simulink model "three_phase_harmonics_pll"  (Simulink 10.3)
settings: Solver=ode23tb  StartTime=0.0  StopTime=0.12  FixedStep=1e-6  MaxStep=1e-4  MinStep=1e-5  RelTol=1e-3  EnableMultiTasking=on
libraries: powerlib_extras x1
settings Model: Creator=ankush  LastModifiedBy=HP
settings DataIOCC: LimitDataPoints=on
settings DebuggingCC: SolverPrmCheckMsg=warning

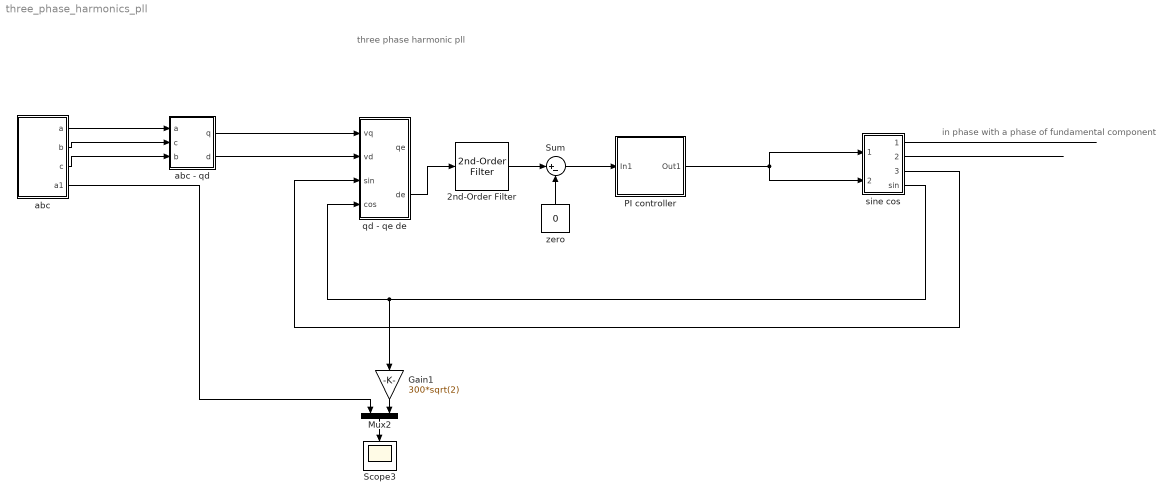
== system three_phase_harmonics_pll ==
  note: in phase with a phase of fundamental component
  note: three phase harmonic pll
  2nd-Order Filter : powerlib_extras/Control  Blocks/2nd-Order Filter  FilterType=Lowpass  Fo=75  Zeta=0.707  Initialize=off  Vac_Init=[1 45 60]  Vdc_Init=-0.5  PlotResponse=off  param1=[1 500 1]
      settings: SourceProductBaseCode=PS
  Gain1 : Gain  Gain=300*sqrt(2)
  Mux2 : Mux  Inputs=2
  PI controller : Subsystem
  Scope3 : Scope
  Sum : Sum  Inputs=|+-
  abc : Subsystem
  abc - qd : Subsystem
  qd - qe de : Subsystem
  sine cos : Subsystem
  zero : Constant  Value=0
  wires:
  abc - qd/1(q) -> qd - qe de/1(vq)
  abc - qd/2(d) -> qd - qe de/2(vd)
  zero/1 -> Sum/2
  sine cos/3(cos) -> qd - qe de/3(sin)
  sine cos/4(sin) -> qd - qe de/4(cos), Gain1/1
  Sum/1 -> PI controller/1(In1)
  PI controller/1(Out1) -> sine cos/1(In1), sine cos/2(In2)
  Mux2/1 -> Scope3/1
  Gain1/1 -> Mux2/2
  abc/2(b) -> abc - qd/2(c)
  abc/1(a) -> abc - qd/1(a)
  abc/3(c) -> abc - qd/3(b)
  qd - qe de/2(de) -> 2nd-Order Filter/1
  2nd-Order Filter/1 -> Sum/1
  abc/4(a1) -> Mux2/1
  sine cos/1(sin1) -> ?
  sine cos/2(cos1) -> ?

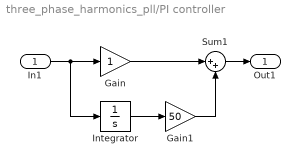
== system three_phase_harmonics_pll/PI controller ==
  In1 : Inport
  Gain : Gain
  Gain1 : Gain  Gain=50
  Integrator : Integrator
  Sum1 : Sum  Inputs=|++
  Out1 : Outport
  wires:
  In1/1 -> Integrator/1, Gain/1
  Integrator/1 -> Gain1/1
  Gain/1 -> Sum1/1
  Gain1/1 -> Sum1/2
  Sum1/1 -> Out1/1

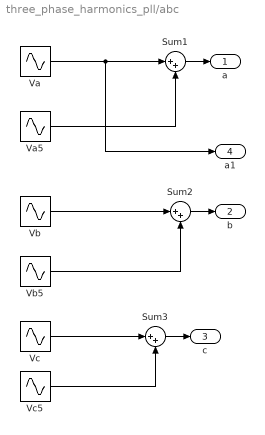
== system three_phase_harmonics_pll/abc ==
  Sum1 : Sum  Inputs=|++
  Sum2 : Sum  Inputs=|++
  Sum3 : Sum  Inputs=|++
  Va : Sin  Amplitude=240*sqrt(2)  Frequency=2*pi*50  SampleTime=0
  Va5 : Sin  Amplitude=50*sqrt(2)  Frequency=2*pi*50*5  SampleTime=0
  Vb : Sin  Amplitude=240*sqrt(2)  Frequency=2*pi*50  Phase=-2*pi/3  SampleTime=0
  Vb5 : Sin  Amplitude=50*sqrt(2)  Frequency=2*pi*50*5  Phase=-2*pi/3  SampleTime=0
  Vc : Sin  Amplitude=240*sqrt(2)  Frequency=2*pi*50  Phase=2*pi/3  SampleTime=0
  Vc5 : Sin  Amplitude=50*sqrt(2)  Frequency=2*pi*50*6  Phase=2*pi/3  SampleTime=0
  a : Outport
  b : Outport  Port=2
  c : Outport  Port=3
  a1 : Outport  Port=4
  wires:
  Va/1 -> Sum1/1, a1/1
  Vb/1 -> Sum2/1
  Vc/1 -> Sum3/1
  Va5/1 -> Sum1/2
  Vb5/1 -> Sum2/2
  Vc5/1 -> Sum3/2
  Sum1/1 -> a/1
  Sum2/1 -> b/1
  Sum3/1 -> c/1

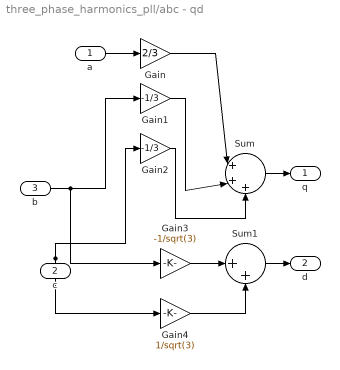
== system three_phase_harmonics_pll/abc - qd ==
  a : Inport
  c : Inport  Port=2
  b : Inport  Port=3
  Gain : Gain  Gain=2/3
  Gain1 : Gain  Gain=-1/3
  Gain2 : Gain  Gain=-1/3
  Gain3 : Gain  Gain=-1/sqrt(3)
  Gain4 : Gain  Gain=1/sqrt(3)
  Sum : Sum  Inputs=|+++
  Sum1 : Sum  Inputs=|++
  q : Outport
  d : Outport  Port=2
  wires:
  Gain/1 -> Sum/1
  Gain1/1 -> Sum/2
  Gain2/1 -> Sum/3
  Gain4/1 -> Sum1/2
  Gain3/1 -> Sum1/1
  a/1 -> Gain/1
  b/1 -> Gain1/1, Gain3/1
  c/1 -> Gain2/1, Gain4/1
  Sum/1 -> q/1
  Sum1/1 -> d/1

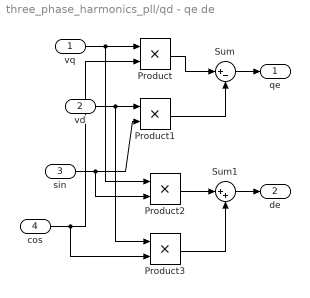
== system three_phase_harmonics_pll/qd - qe de ==
  vq : Inport
  vd : Inport  Port=2
  sin : Inport  Port=3
  cos : Inport  Port=4
  Product{,1..3} (4 alike) : Product  RndMeth=Zero
  Sum : Sum  Inputs=|+-
  Sum1 : Sum  Inputs=|++
  qe : Outport
  de : Outport  Port=2
  wires:
  cos/1 -> Product3/2, Product/2
  sin/1 -> Product2/2, Product1/2
  Product/1 -> Sum/1
  Product1/1 -> Sum/2
  Product2/1 -> Sum1/1
  Product3/1 -> Sum1/2
  vq/1 -> Product/1, Product2/1
  vd/1 -> Product1/1, Product3/1
  Sum/1 -> qe/1
  Sum1/1 -> de/1

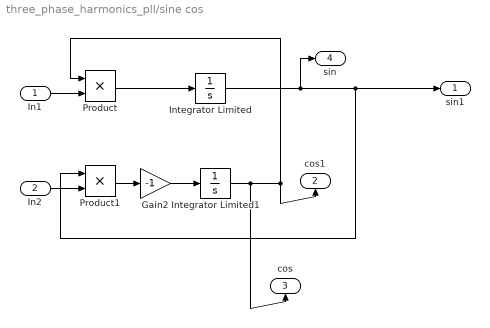
== system three_phase_harmonics_pll/sine cos ==
  In1 : Inport
  In2 : Inport  Port=2
  Gain2 : Gain  Gain=-1
  Integrator Limited : Integrator  InitialCondition=1  LimitOutput=on  UpperSaturationLimit=1  LowerSaturationLimit=-1
  Integrator Limited1 : Integrator  LimitOutput=on  UpperSaturationLimit=1  LowerSaturationLimit=-1
  Product : Product  RndMeth=Zero
  Product1 : Product  RndMeth=Zero
  sin1 : Outport
  cos1 : Outport  Port=2
  cos : Outport  Port=3
  sin : Outport  Port=4
  wires:
  Product/1 -> Integrator Limited/1
  Integrator Limited1/1 -> Product/1, cos1/1, cos/1
  Product1/1 -> Gain2/1
  Gain2/1 -> Integrator Limited1/1
  Integrator Limited/1 -> sin/1, Product1/1, sin1/1
  In1/1 -> Product/2
  In2/1 -> Product1/2
